simulink model "A"  (R2023b)
settings: Solver=VariableStepAuto  StartTime=0.0  StopTime=10.0  RelTol=1e-3
settings Model: Creator=jakub  LastModifiedBy=jakub

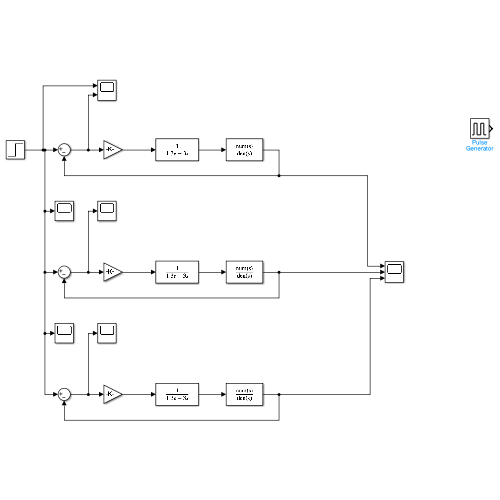
[thumbnail: Simulink's stored preview of the top-level diagram]
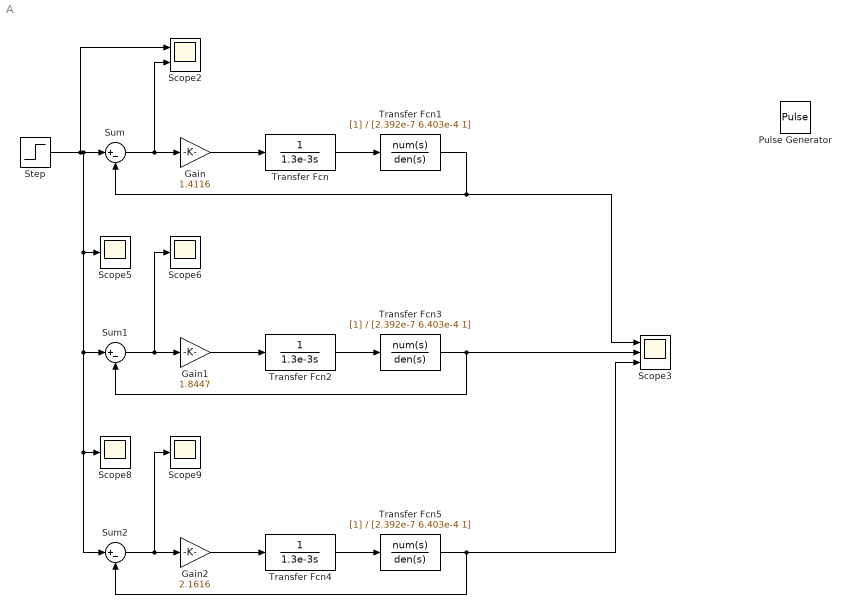
== system A ==
  Gain : Gain  Gain=1.4116
  Gain1 : Gain  Gain=1.8447
  Gain2 : Gain  Gain=2.1616
  Pulse Generator : DiscretePulseGenerator  PulseType=Time based  Period=0.1  PulseWidth=50
  Scope2 : Scope  NumInputPorts=2
  Scope3 : Scope  NumInputPorts=3
  Scope{5..6,8..9} (4 alike) : Scope
  Step : Step  SampleTime=0
  Sum : Sum  Inputs=|+-
  Sum1 : Sum  Inputs=|+-
  Sum2 : Sum  Inputs=|+-
  Transfer Fcn : TransferFcn  Denominator=[1.3e-3 0]
  Transfer Fcn1 : TransferFcn  Denominator=[2.392e-7 6.403e-4 1]
  Transfer Fcn2 : TransferFcn  Denominator=[1.3e-3 0]
  Transfer Fcn3 : TransferFcn  Denominator=[2.392e-7 6.403e-4 1]
  Transfer Fcn4 : TransferFcn  Denominator=[1.3e-3 0]
  Transfer Fcn5 : TransferFcn  Denominator=[2.392e-7 6.403e-4 1]
  wires:
  Sum/1 -> Scope2/2, Gain/1
  Gain/1 -> Transfer Fcn/1
  Transfer Fcn/1 -> Transfer Fcn1/1
  Transfer Fcn1/1 -> Scope3/1, Sum/2
  Transfer Fcn3/1 -> Sum1/2, Scope3/2
  Sum1/1 -> Scope6/1, Gain1/1
  Gain1/1 -> Transfer Fcn2/1
  Transfer Fcn2/1 -> Transfer Fcn3/1
  Step/1 -> Sum2/1, Scope8/1, Sum1/1, Scope5/1, Sum/1, Scope2/1
  Transfer Fcn5/1 -> Scope3/3, Sum2/2
  Sum2/1 -> Scope9/1, Gain2/1
  Gain2/1 -> Transfer Fcn4/1
  Transfer Fcn4/1 -> Transfer Fcn5/1
